simulink model "const_in_subsystem"  (R2023a)
settings: Solver=VariableStepAuto  StartTime=0.0  StopTime=10.0  RelTol=1e-3
settings Model: Creator=Martin  LastModifiedBy=Martin
settings ModelReferenceCC: EnableRefExpFcnMdlSchedulingChecks=on

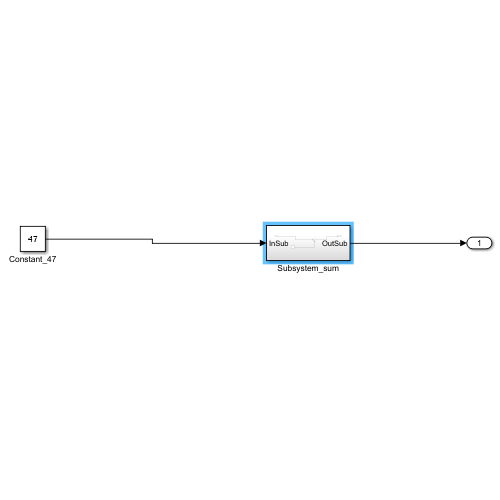
[thumbnail: Simulink's stored preview of the top-level diagram]
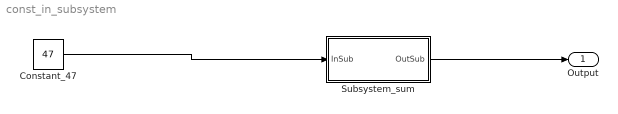
== system const_in_subsystem ==
  Constant_47 : Constant  Value=47
  Subsystem_sum : Subsystem
  Output : Outport
  wires:
  Subsystem_sum/1(OutSub) -> Output/1
  Constant_47/1 -> Subsystem_sum/1(InSub)

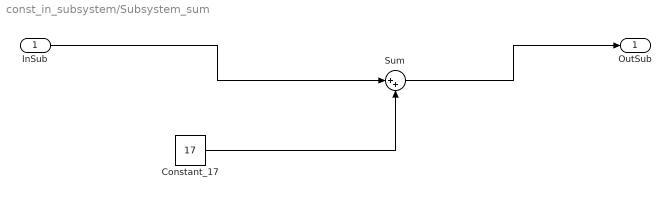
== system const_in_subsystem/Subsystem_sum ==
  InSub : Inport
  Constant_17 : Constant  Value=17
  Sum : Sum  Inputs=|++
  OutSub : Outport
  wires:
  InSub/1 -> Sum/1
  Sum/1 -> OutSub/1
  Constant_17/1 -> Sum/2
